simulink model "essai_echelon_volt"  (R2024a)
settings: Solver=VariableStepAuto  StartTime=0.0  StopTime=1000  RelTol=1e-3
InitFcn:
  | step_initial = get_param('simulink16marshihi/Échelon', 'Before');
  | set_param('simulink16marshihi/Température initiale', 'Value', step_initial);
  | set_param('simulink16marshihi/Chauffage/po_chauffage', 'Value', step_initial);
  | set_param('simulink16marshihi/Refroidissement/po_refroidissement', 'Value', step_initial);
  | consigne = get_param('simulink16marshihi/Échelon', 'After');
  | consigne = str2double(consigne);
  | step_initial = str2double(step_initial);
  | five_up = consigne + 0.05*abs(consigne-step_initial);
  | five_down = consigne - 0.05*abs(consigne-step_initial);
  | set_param('simulink16marshihi/+5%', 'Value', num2str(five_up));
  | set_param('simulink16marshihi/-5%', 'Value', num2str(five_down));
settings Model: Creator=sabri  LastModifiedBy=MADER143

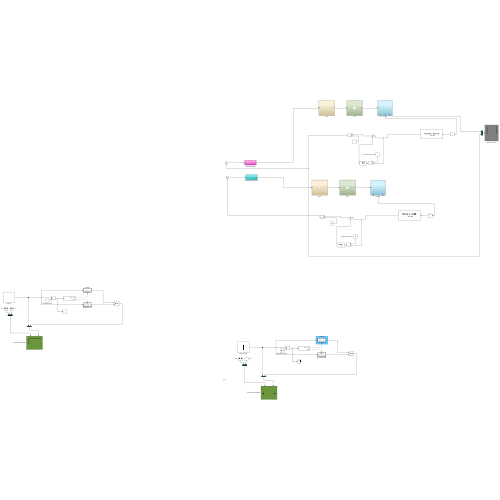
[thumbnail: Simulink's stored preview of the top-level diagram]
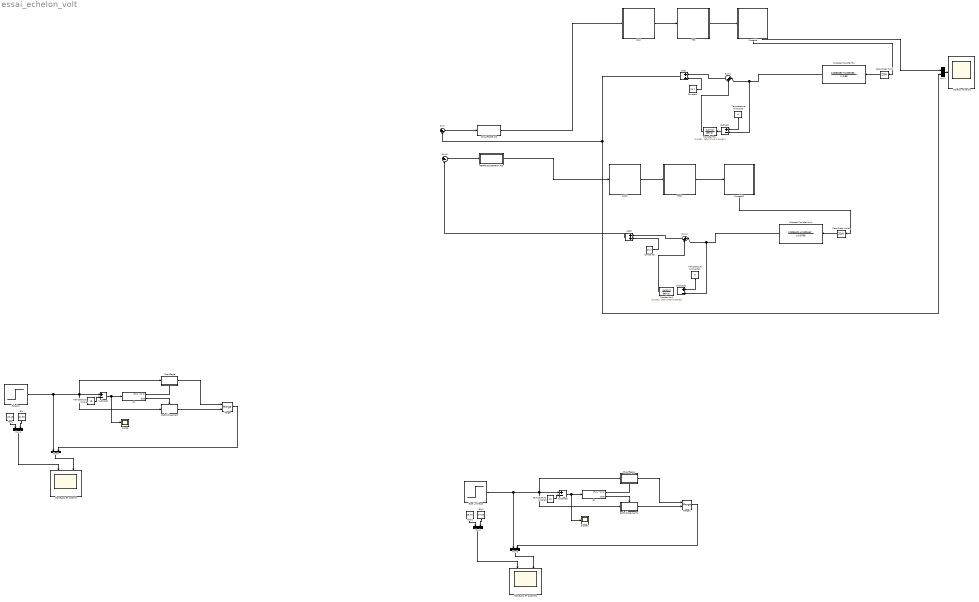
== system essai_echelon_volt ==
  " ÉCHELON ET SORTIE" : Scope  NumInputPorts=2
  " ÉCHELON ET SORTIE1" : Scope  NumInputPorts=2
  +5% : Constant  Value=25.45
  +5%1 : Constant  Value=25.45
  -5% : Constant  Value=24.55
  -5%1 : Constant  Value=24.55
  Add1 : Sum
  Add2 : Sum
  CHAUFFAGE PID : Subsystem
  Chauffage : Subsystem  TreatAsAtomicUnit=on
  Chauffage1 : Subsystem  TreatAsAtomicUnit=on
  Constant : Constant  Value=23.7
  Constant3 : Constant  Value=23.7
  DAC : Subsystem
  DAC1 : Subsystem
  Discrete Transfer Fcn : DiscreteTransferFcn  Numerator=[0.009158 0.009158]  Denominator=[1 -0.98]
  Discrete Transfer Fcn1 : DiscreteTransferFcn  Numerator=[0.009442 0.009442]  Denominator=[1 -0.9796]
  Essai_voltage : Step  Time=0  Before=16  After=25  SampleTime=0
  If1 : If  IfExpression=u1 >= 0
  If2 : If  IfExpression=u1 >= 0
  Merge : Merge
  Merge1 : Merge
  Mux{1..5} (5 alike) : Mux  Inputs=2
  Procédé : Subsystem
      settings: PortSchema="{\"entries\":[{\"content\":{\"sides\":[{\"content\":{\"connectorIds\":[\"In1\"]},\"type\":\"ConnectorPlacement.EquallySpacedRectSide\",\"uuid\":\"20a23230-a41b-4fdf-8ae4-039aa17abee7\"},{\"content\":{\"side\":\"RIGHT\"},\"type\":\"ConnectorPlacement.EquallySpacedRectSide\",\"uuid\":\"82e4e468-e0ad-4c9f-b6ff-cc9c1ee7ea9d\"},{\"content\":{\"side\":\"TOP\"},\"type\":\"ConnectorPlacement.EquallySpacedRectSide\",\"uuid\":\"049bc4af-9a9a-43aa-9803-dca862d69d2b\"},{\"content\":{\"connectorIds\":[\"Out1\",\"Out2\",\"Out3\"],\"side\":\"BOTTOM\"},\"type\":\"ConnectorPlacement.EquallySpacedRectSide\",\"uuid\":\"142d2b37-1c32-477b-9e70-4e4bc8b2913e\"}]},\"type\":\"ConnectorPlacement.EquallySpacedConnector\",\"uuid\":\"a0abf580-2deb-4a1c-9cb8-1272669a26fd\"}],\"packageUris\":[\"http://schema.mathworks.com/mf0/Connector/R2020b\"],\"version\":\"1.0\"}"
  Procédé1 : Subsystem
      settings: PortSchema="{\"entries\":[{\"content\":{\"sides\":[{\"content\":{\"connectorIds\":[\"In1\"]},\"type\":\"ConnectorPlacement.EquallySpacedRectSide\",\"uuid\":\"20a23230-a41b-4fdf-8ae4-039aa17abee7\"},{\"content\":{\"side\":\"RIGHT\"},\"type\":\"ConnectorPlacement.EquallySpacedRectSide\",\"uuid\":\"82e4e468-e0ad-4c9f-b6ff-cc9c1ee7ea9d\"},{\"content\":{\"side\":\"TOP\"},\"type\":\"ConnectorPlacement.EquallySpacedRectSide\",\"uuid\":\"049bc4af-9a9a-43aa-9803-dca862d69d2b\"},{\"content\":{\"connectorIds\":[\"Out1\",\"Out2\",\"Out3\"],\"side\":\"BOTTOM\"},\"type\":\"ConnectorPlacement.EquallySpacedRectSide\",\"uuid\":\"142d2b37-1c32-477b-9e70-4e4bc8b2913e\"}]},\"type\":\"ConnectorPlacement.EquallySpacedConnector\",\"uuid\":\"a0abf580-2deb-4a1c-9cb8-1272669a26fd\"}],\"packageUris\":[\"http://schema.mathworks.com/mf0/Connector/R2020b\"],\"version\":\"1.0\"}"
  REFROIDISSEMENT PID : Subsystem
  Refroidissement : Subsystem  TreatAsAtomicUnit=on
  Refroidissement1 : Subsystem  TreatAsAtomicUnit=on
  Scope : Scope
  Scope1 : Scope
  Subtract{,1..3} (4 alike) : Sum  Inputs=+-
  Sum : Sum  Inputs=|+-
  Sum1 : Sum  Inputs=|++
  Sum2 : Sum  Inputs=|++
  Sum3 : Sum  Inputs=|+-
  TEC : Subsystem
  TEC1 : Subsystem
  Température ambiante : Constant  Value=0
  Température ambiante1 : Constant  Value=0
  Température initiale : Constant  Value=16
  Température initiale1 : Constant  Value=16
  Transfer Fcn : TransferFcn  Numerator=[13.65]  Denominator=[900*2700*0.00161]
  Transfer Fcn1 : TransferFcn  Numerator=[13.65]  Denominator=[900*2700*0.00161]
  Zero-Order Hold : ZeroOrderHold  SampleTime=0.5
  Zero-Order Hold1 : ZeroOrderHold  SampleTime=0.5
  Échelon : Step  Time=0  Before=16  After=25  SampleTime=0
  Échelon et sortie : Scope
  wires:
  Échelon/1 -> Chauffage/1(In1), Subtract2/1, Refroidissement/1(In1), Mux5/1
  ? -> ?
  Température initiale/1 -> Subtract2/2
  +5%/1 -> Mux4/1
  -5%/1 -> Mux4/2
  If1/1 -> Chauffage/Action
  If1/2 -> Refroidissement/Action
  TEC1/1(W) -> Procédé1/1(W)
  DAC1/1(V) -> TEC1/1(V)
  Procédé1/2(y2) -> Zero-Order Hold1/1
  Température ambiante1/1 -> Subtract1/1
  Sum/1 -> CHAUFFAGE PID/1(In1)
  Sum2/1 -> Add2/1
  Add2/1 -> Sum3/2
  Sum3/1 -> REFROIDISSEMENT PID/1(In1)
  REFROIDISSEMENT PID/1(dc) -> DAC1/1(dc)
  Transfer Fcn1/1 -> Sum2/2
  Zero-Order Hold1/1 -> Discrete Transfer Fcn1/1
  Add1/1 -> Sum/2, Mux1/2
  Procédé/2(y2) -> Zero-Order Hold/1
  Zero-Order Hold/1 -> Discrete Transfer Fcn/1
  Subtract/1 -> Transfer Fcn/1
  Constant/1 -> Add1/2
  Discrete Transfer Fcn1/1 -> Sum2/1, Subtract1/2
  TEC/1(W) -> Procédé/1(W)
  CHAUFFAGE PID/1(dc) -> DAC/1(dc)
  Discrete Transfer Fcn/1 -> Sum1/1, Subtract/2
  Transfer Fcn/1 -> Sum1/2
  DAC/1(V) -> TEC/1(V)
  Sum1/1 -> Add1/1
  Constant3/1 -> Add2/2
  Procédé/3(y3) -> Mux1/1
  Température ambiante/1 -> Subtract/1
  Mux1/1 -> Échelon et sortie/1
  Chauffage/1(Out1) -> Merge/1
  Refroidissement/1(Out1) -> Merge/2
  Merge/1 -> Mux5/2
  Subtract2/1 -> Scope/1, If1/1
  Mux5/1 -> " ÉCHELON ET SORTIE"/2
  Mux4/1 -> " ÉCHELON ET SORTIE"/1
  Mux2/1 -> " ÉCHELON ET SORTIE1"/1
  Chauffage1/1(Out1) -> Merge1/1
  Mux3/1 -> " ÉCHELON ET SORTIE1"/2
  Refroidissement1/1(Out1) -> Merge1/2
  Merge1/1 -> Mux3/2
  Subtract3/1 -> Scope1/1, If2/1
  If2/2 -> Refroidissement1/Action
  If2/1 -> Chauffage1/Action
  +5%1/1 -> Mux2/1
  Température initiale1/1 -> Subtract3/2
  -5%1/1 -> Mux2/2
  Essai_voltage/1 -> Chauffage1/1(In1), Subtract3/1, Refroidissement1/1(In1), Mux3/1

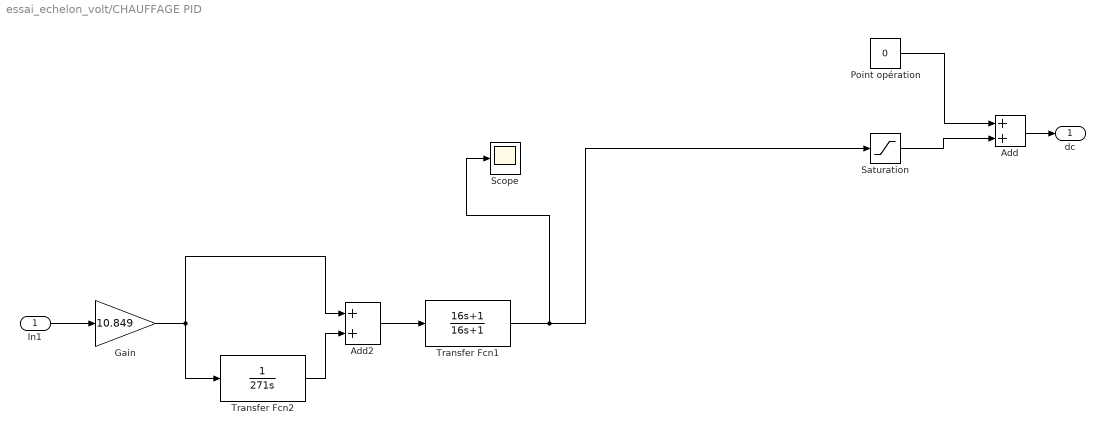
== system essai_echelon_volt/CHAUFFAGE PID ==
  In1 : Inport
  Add : Sum
  Add2 : Sum
  Gain : Gain  Gain=10.849
  Point opération : Constant  Value=0
  Saturation : Saturate  UpperLimit=255  LowerLimit=-255
  Scope : Scope
  Transfer Fcn1 : TransferFcn  Numerator=[16 1]  Denominator=[16 1]
  Transfer Fcn2 : TransferFcn  Denominator=[271 0]
  dc : Outport
  wires:
  Add2/1 -> Transfer Fcn1/1
  Saturation/1 -> Add/2
  Point opération/1 -> Add/1
  Transfer Fcn1/1 -> Scope/1, Saturation/1
  Gain/1 -> Transfer Fcn2/1, Add2/1
  Transfer Fcn2/1 -> Add2/2
  In1/1 -> Gain/1
  Add/1 -> dc/1

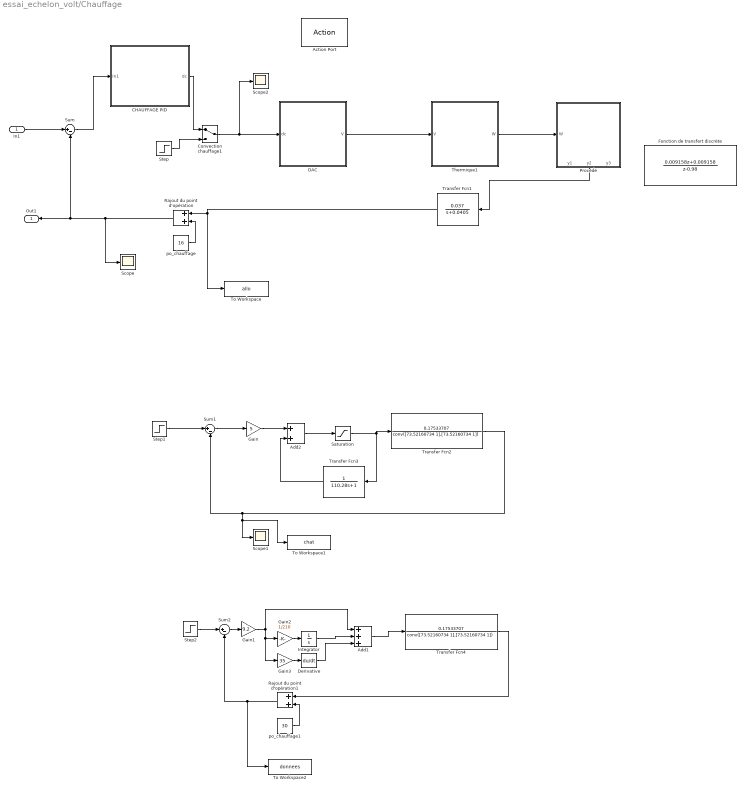
== system essai_echelon_volt/Chauffage ==
  In1 : Inport
  Action Port : ActionPort  ActionPortLabel=if(u1 >= 0)
  Add1 : Sum  Inputs=+++
  Add2 : Sum
  CHAUFFAGE PID : Subsystem
  Convection chauffage1 : ManualSwitch
  DAC : Subsystem
  Derivative : Derivative
  Fonction de transfert discrète : DiscreteTransferFcn  Numerator=[0.009158 0.009158]  Denominator=[1 -0.98]
  Gain : Gain  Gain=5
  Gain1 : Gain  Gain=9.2
  Gain2 : Gain  Gain=1/210
  Gain3 : Gain  Gain=35
  Integrator : Integrator
  Procédé : Subsystem
      settings: PortSchema="{\"entries\":[{\"content\":{\"sides\":[{\"content\":{\"connectorIds\":[\"In1\"]},\"type\":\"ConnectorPlacement.EquallySpacedRectSide\",\"uuid\":\"20a23230-a41b-4fdf-8ae4-039aa17abee7\"},{\"content\":{\"side\":\"RIGHT\"},\"type\":\"ConnectorPlacement.EquallySpacedRectSide\",\"uuid\":\"82e4e468-e0ad-4c9f-b6ff-cc9c1ee7ea9d\"},{\"content\":{\"side\":\"TOP\"},\"type\":\"ConnectorPlacement.EquallySpacedRectSide\",\"uuid\":\"049bc4af-9a9a-43aa-9803-dca862d69d2b\"},{\"content\":{\"connectorIds\":[\"Out1\",\"Out2\",\"Out3\"],\"side\":\"BOTTOM\"},\"type\":\"ConnectorPlacement.EquallySpacedRectSide\",\"uuid\":\"142d2b37-1c32-477b-9e70-4e4bc8b2913e\"}]},\"type\":\"ConnectorPlacement.EquallySpacedConnector\",\"uuid\":\"a0abf580-2deb-4a1c-9cb8-1272669a26fd\"}],\"packageUris\":[\"http://schema.mathworks.com/mf0/Connector/R2020b\"],\"version\":\"1.0\"}"
  Rajout du point d'opération : Sum
  Rajout du point d'opération1 : Sum
  Saturation : Saturate  UpperLimit=100  LowerLimit=-100
  Scope : Scope
  Scope1 : Scope
  Scope2 : Scope
  Step : Step  Time=0  After=20  SampleTime=0
  Step1 : Step  Time=0  After=7  SampleTime=0
  Step2 : Step  Time=0  Before=23  After=30  SampleTime=0
  Sum : Sum  Inputs=|+-
  Sum1 : Sum  Inputs=|+-
  Sum2 : Sum  Inputs=|+-
  Thermique1 : Subsystem
  To Workspace : ToWorkspace  VariableName=allo  SampleTime=-1
  To Workspace1 : ToWorkspace  VariableName=chat  SampleTime=-1
  To Workspace2 : ToWorkspace  VariableName=donnees  SampleTime=-1
  Transfer Fcn1 : TransferFcn  Numerator=[0.037]  Denominator=[1 0.0405]
  Transfer Fcn2 : TransferFcn  Numerator=[0.17533707]  Denominator=conv([73.52160734 1],[73.52160734 1])
  Transfer Fcn3 : TransferFcn  Denominator=[110.28 1]
  Transfer Fcn4 : TransferFcn  Numerator=[0.17533707]  Denominator=conv([73.52160734 1],[73.52160734 1])
  po_chauffage : Constant  Value=16
  po_chauffage1 : Constant  Value=30
  Out1 : Outport
  wires:
  Sum/1 -> CHAUFFAGE PID/1(In1)
  In1/1 -> Sum/1
  Rajout du point d'opération/1 -> Scope/1, Out1/1, Sum/2
  po_chauffage/1 -> Rajout du point d'opération/2
  Procédé/2(y2) -> Transfer Fcn1/1
  Transfer Fcn1/1 -> To Workspace/1, Rajout du point d'opération/1
  DAC/1(V) -> Thermique1/1(V)
  CHAUFFAGE PID/1(dc) -> Convection chauffage1/1
  Convection chauffage1/1 -> Scope2/1, DAC/1(dc)
  Step/1 -> Convection chauffage1/2
  Step1/1 -> Sum1/1
  Transfer Fcn2/1 -> To Workspace1/1, Scope1/1, Sum1/2
  Gain/1 -> Add2/1
  Transfer Fcn3/1 -> Add2/2
  Add2/1 -> Saturation/1
  Saturation/1 -> Transfer Fcn2/1, Transfer Fcn3/1
  Sum1/1 -> Gain/1
  Thermique1/1(W) -> Procédé/1(W)
  Gain2/1 -> Integrator/1
  Add1/1 -> Transfer Fcn4/1
  Gain3/1 -> Derivative/1
  Sum2/1 -> Gain1/1
  Integrator/1 -> Add1/2
  Derivative/1 -> Add1/3
  Gain1/1 -> Add1/1, Gain3/1, Gain2/1
  Rajout du point d'opération1/1 -> To Workspace2/1, Sum2/2
  Transfer Fcn4/1 -> Rajout du point d'opération1/1
  po_chauffage1/1 -> Rajout du point d'opération1/2
  Step2/1 -> Sum2/1

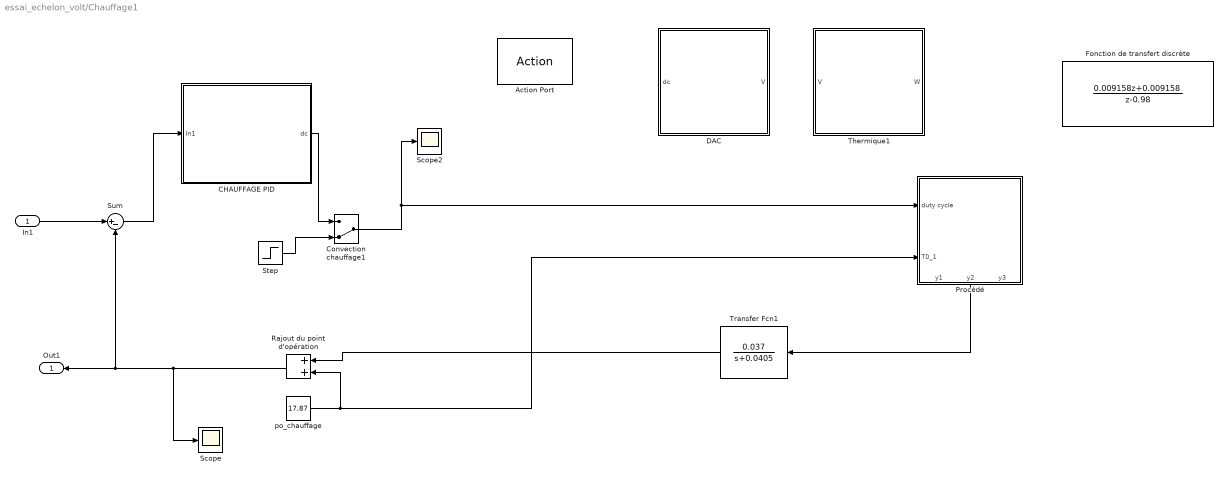
== system essai_echelon_volt/Chauffage1 ==
  In1 : Inport
  Action Port : ActionPort  ActionPortLabel=if(u1 >= 0)
  CHAUFFAGE PID : Subsystem
  Convection chauffage1 : ManualSwitch  CurrentSetting=0
  DAC : Subsystem
  Fonction de transfert discrète : DiscreteTransferFcn  Numerator=[0.009158 0.009158]  Denominator=[1 -0.98]
  Procédé : Subsystem
      settings: PortSchema="{\"entries\":[{\"content\":{\"sides\":[{\"content\":{\"connectorIds\":[\"In1\",\"In2\"]},\"type\":\"ConnectorPlacement.EquallySpacedRectSide\",\"uuid\":\"20a23230-a41b-4fdf-8ae4-039aa17abee7\"},{\"content\":{\"side\":\"RIGHT\"},\"type\":\"ConnectorPlacement.EquallySpacedRectSide\",\"uuid\":\"82e4e468-e0ad-4c9f-b6ff-cc9c1ee7ea9d\"},{\"content\":{\"side\":\"TOP\"},\"type\":\"ConnectorPlacement.EquallySpacedRectSide\",\"uuid\":\"049bc4af-9a9a-43aa-9803-dca862d69d2b\"},{\"content\":{\"connectorIds\":[\"Out1\",\"Out2\",\"Out3\"],\"side\":\"BOTTOM\"},\"type\":\"ConnectorPlacement.EquallySpacedRectSide\",\"uuid\":\"142d2b37-1c32-477b-9e70-4e4bc8b2913e\"}]},\"type\":\"ConnectorPlacement.EquallySpacedConnector\",\"uuid\":\"a0abf580-2deb-4a1c-9cb8-1272669a26fd\"}],\"packageUris\":[\"http://schema.mathworks.com/mf0/Connector/R2020b\"],\"version\":\"1.0\"}"
  Rajout du point d'opération : Sum
  Scope : Scope
  Scope2 : Scope
  Step : Step  Time=0  After=3.92  SampleTime=0
  Sum : Sum  Inputs=|+-
  Thermique1 : Subsystem
  Transfer Fcn1 : TransferFcn  Numerator=[0.037]  Denominator=[1 0.0405]
  po_chauffage : Constant  Value=17.87
  Out1 : Outport
  wires:
  Sum/1 -> CHAUFFAGE PID/1(In1)
  In1/1 -> Sum/1
  Rajout du point d'opération/1 -> Scope/1, Out1/1, Sum/2
  po_chauffage/1 -> Procédé/2(T0_1), Rajout du point d'opération/2
  Procédé/2(y2) -> Transfer Fcn1/1
  Transfer Fcn1/1 -> Rajout du point d'opération/1
  CHAUFFAGE PID/1(dc) -> Convection chauffage1/1
  Convection chauffage1/1 -> Procédé/1(duty cycle), Scope2/1
  Step/1 -> Convection chauffage1/2

== system essai_echelon_volt/DAC ==
  dc : Inport
  Slope : Gain  Gain=0.079
  V : Outport
  wires:
  dc/1 -> Slope/1
  Slope/1 -> V/1

== system essai_echelon_volt/DAC1 ==
  dc : Inport
  Slope : Gain  Gain=0.079
  V : Outport
  wires:
  dc/1 -> Slope/1
  Slope/1 -> V/1

== system essai_echelon_volt/Procédé ==
  W : Inport
  Add : Sum
  G1 : TransferFcn  Numerator=[0.006923]  Denominator=[1 0.01236]
  G2 : TransferFcn  Numerator=[0.01782]  Denominator=[1 0.02491]
  G3 : TransferFcn  Numerator=[0.037]  Denominator=[1 0.0405]
  Step : Step  Time=60  After=0  SampleTime=0
  y1 : Outport
  y2 : Outport  Port=2
  y3 : Outport  Port=3
  wires:
  G1/1 -> y1/1, G2/1
  Add/1 -> G1/1
  W/1 -> Add/1
  Step/1 -> Add/2
  G2/1 -> G3/1, y2/1
  G3/1 -> y3/1

== system essai_echelon_volt/Procédé1 ==
  W : Inport
  Add : Sum
  G1 : TransferFcn  Numerator=[0.009117]  Denominator=[1 0.01046]
  G2 : TransferFcn  Numerator=[0.03203]  Denominator=[1 0.03834]
  G3 : TransferFcn  Numerator=[0.03816]  Denominator=[1 0.04131]
  Step : Step  Time=60  After=0  SampleTime=0
  y1 : Outport
  y2 : Outport  Port=2
  y3 : Outport  Port=3
  wires:
  G1/1 -> y1/1, G2/1
  Add/1 -> G1/1
  W/1 -> Add/1
  Step/1 -> Add/2
  G2/1 -> G3/1, y2/1
  G3/1 -> y3/1

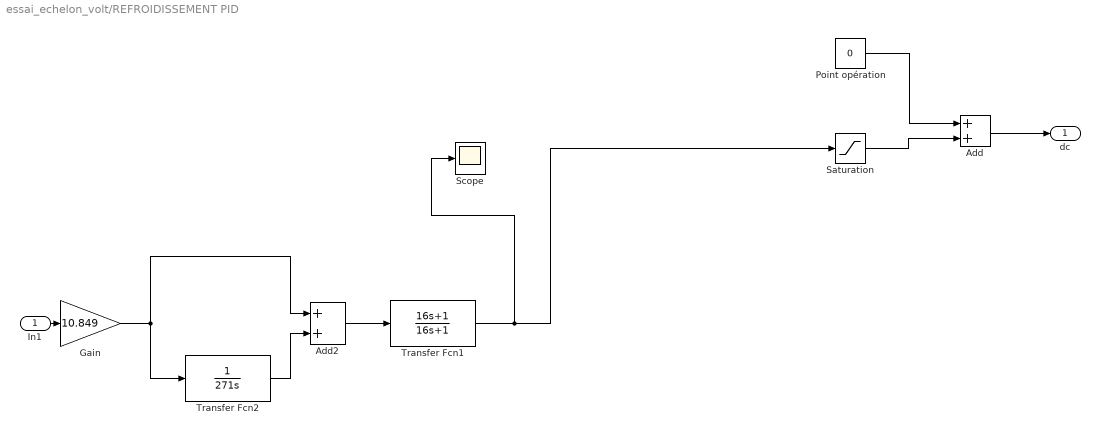
== system essai_echelon_volt/REFROIDISSEMENT PID ==
  In1 : Inport
  Add : Sum
  Add2 : Sum
  Gain : Gain  Gain=10.849
  Point opération : Constant  Value=0
  Saturation : Saturate  UpperLimit=255  LowerLimit=-255
  Scope : Scope
  Transfer Fcn1 : TransferFcn  Numerator=[16 1]  Denominator=[16 1]
  Transfer Fcn2 : TransferFcn  Denominator=[271 0]
  dc : Outport
  wires:
  Add2/1 -> Transfer Fcn1/1
  Saturation/1 -> Add/2
  Point opération/1 -> Add/1
  Transfer Fcn1/1 -> Scope/1, Saturation/1
  Gain/1 -> Transfer Fcn2/1, Add2/1
  Transfer Fcn2/1 -> Add2/2
  In1/1 -> Gain/1
  Add/1 -> dc/1

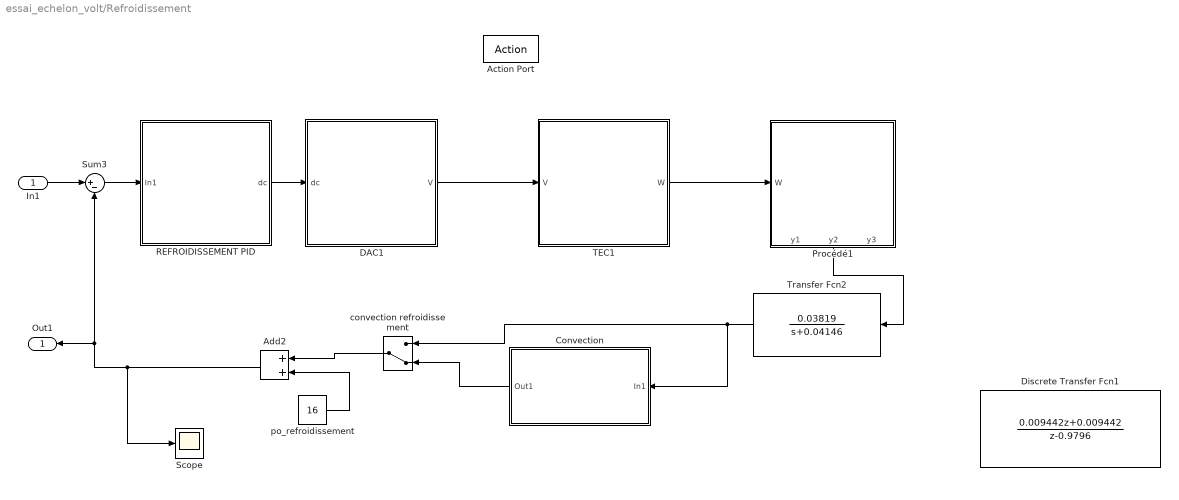
== system essai_echelon_volt/Refroidissement ==
  In1 : Inport
  Action Port : ActionPort  ActionPortLabel=else
  Add2 : Sum
  Convection : Subsystem
  DAC1 : Subsystem
  Discrete Transfer Fcn1 : DiscreteTransferFcn  Numerator=[0.009442 0.009442]  Denominator=[1 -0.9796]
  Procédé1 : Subsystem
      settings: PortSchema="{\"entries\":[{\"content\":{\"sides\":[{\"content\":{\"connectorIds\":[\"In1\"]},\"type\":\"ConnectorPlacement.EquallySpacedRectSide\",\"uuid\":\"20a23230-a41b-4fdf-8ae4-039aa17abee7\"},{\"content\":{\"side\":\"RIGHT\"},\"type\":\"ConnectorPlacement.EquallySpacedRectSide\",\"uuid\":\"82e4e468-e0ad-4c9f-b6ff-cc9c1ee7ea9d\"},{\"content\":{\"side\":\"TOP\"},\"type\":\"ConnectorPlacement.EquallySpacedRectSide\",\"uuid\":\"049bc4af-9a9a-43aa-9803-dca862d69d2b\"},{\"content\":{\"connectorIds\":[\"Out1\",\"Out2\",\"Out3\"],\"side\":\"BOTTOM\"},\"type\":\"ConnectorPlacement.EquallySpacedRectSide\",\"uuid\":\"142d2b37-1c32-477b-9e70-4e4bc8b2913e\"}]},\"type\":\"ConnectorPlacement.EquallySpacedConnector\",\"uuid\":\"a0abf580-2deb-4a1c-9cb8-1272669a26fd\"}],\"packageUris\":[\"http://schema.mathworks.com/mf0/Connector/R2020b\"],\"version\":\"1.0\"}"
  REFROIDISSEMENT PID : Subsystem
  Scope : Scope
  Sum3 : Sum  Inputs=|+-
  TEC1 : Subsystem
  Transfer Fcn2 : TransferFcn  Numerator=[0.03819]  Denominator=[1 0.04146]
  convection refroidissement : ManualSwitch  CurrentSetting=0
  po_refroidissement : Constant  Value=16
  Out1 : Outport
  wires:
  TEC1/1(W) -> Procédé1/1(W)
  DAC1/1(V) -> TEC1/1(V)
  Procédé1/2(y2) -> Transfer Fcn2/1
  po_refroidissement/1 -> Add2/2
  Add2/1 -> Scope/1, Out1/1, Sum3/2
  Sum3/1 -> REFROIDISSEMENT PID/1(In1)
  REFROIDISSEMENT PID/1(dc) -> DAC1/1(dc)
  In1/1 -> Sum3/1
  Transfer Fcn2/1 -> Convection/1(In1), convection refroidissement/1
  convection refroidissement/1 -> Add2/1
  Convection/1(Out1) -> convection refroidissement/2

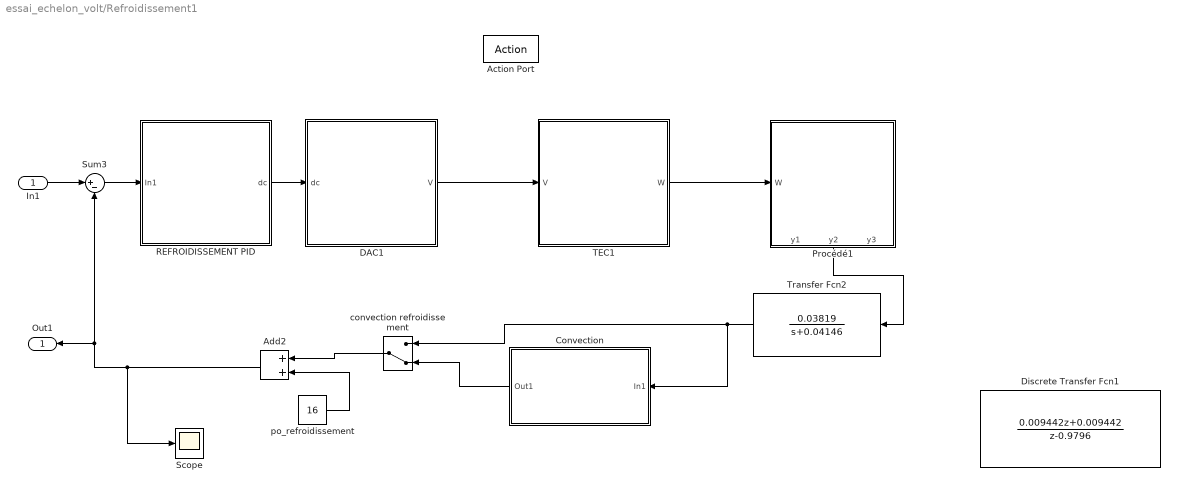
== system essai_echelon_volt/Refroidissement1 ==
  In1 : Inport
  Action Port : ActionPort  ActionPortLabel=else
  Add2 : Sum
  Convection : Subsystem
  DAC1 : Subsystem
  Discrete Transfer Fcn1 : DiscreteTransferFcn  Numerator=[0.009442 0.009442]  Denominator=[1 -0.9796]
  Procédé1 : Subsystem
      settings: PortSchema="{\"entries\":[{\"content\":{\"sides\":[{\"content\":{\"connectorIds\":[\"In1\"]},\"type\":\"ConnectorPlacement.EquallySpacedRectSide\",\"uuid\":\"20a23230-a41b-4fdf-8ae4-039aa17abee7\"},{\"content\":{\"side\":\"RIGHT\"},\"type\":\"ConnectorPlacement.EquallySpacedRectSide\",\"uuid\":\"82e4e468-e0ad-4c9f-b6ff-cc9c1ee7ea9d\"},{\"content\":{\"side\":\"TOP\"},\"type\":\"ConnectorPlacement.EquallySpacedRectSide\",\"uuid\":\"049bc4af-9a9a-43aa-9803-dca862d69d2b\"},{\"content\":{\"connectorIds\":[\"Out1\",\"Out2\",\"Out3\"],\"side\":\"BOTTOM\"},\"type\":\"ConnectorPlacement.EquallySpacedRectSide\",\"uuid\":\"142d2b37-1c32-477b-9e70-4e4bc8b2913e\"}]},\"type\":\"ConnectorPlacement.EquallySpacedConnector\",\"uuid\":\"a0abf580-2deb-4a1c-9cb8-1272669a26fd\"}],\"packageUris\":[\"http://schema.mathworks.com/mf0/Connector/R2020b\"],\"version\":\"1.0\"}"
  REFROIDISSEMENT PID : Subsystem
  Scope : Scope
  Sum3 : Sum  Inputs=|+-
  TEC1 : Subsystem
  Transfer Fcn2 : TransferFcn  Numerator=[0.03819]  Denominator=[1 0.04146]
  convection refroidissement : ManualSwitch  CurrentSetting=0
  po_refroidissement : Constant  Value=16
  Out1 : Outport
  wires:
  TEC1/1(W) -> Procédé1/1(W)
  DAC1/1(V) -> TEC1/1(V)
  Procédé1/2(y2) -> Transfer Fcn2/1
  po_refroidissement/1 -> Add2/2
  Add2/1 -> Scope/1, Out1/1, Sum3/2
  Sum3/1 -> REFROIDISSEMENT PID/1(In1)
  REFROIDISSEMENT PID/1(dc) -> DAC1/1(dc)
  In1/1 -> Sum3/1
  Transfer Fcn2/1 -> Convection/1(In1), convection refroidissement/1
  convection refroidissement/1 -> Add2/1
  Convection/1(Out1) -> convection refroidissement/2

== system essai_echelon_volt/TEC ==
  V : Inport
  MATLAB Function : MATLAB Function  TreatAsAtomicUnit=on
  W : Outport
  wires:
  V/1 -> MATLAB Function/1(u)
  MATLAB Function/1(y) -> W/1

== system essai_echelon_volt/TEC1 ==
  V : Inport
  MATLAB Function : MATLAB Function  TreatAsAtomicUnit=on
  W : Outport
  wires:
  V/1 -> MATLAB Function/1(u)
  MATLAB Function/1(y) -> W/1

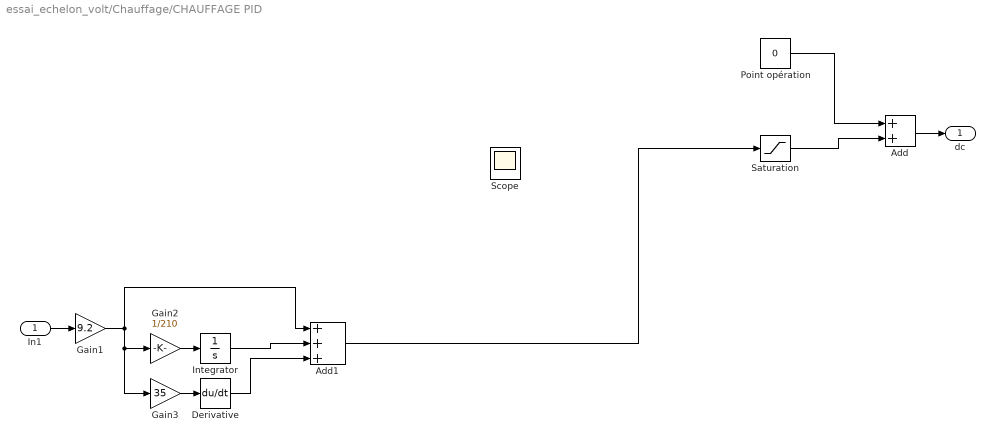
== system essai_echelon_volt/Chauffage/CHAUFFAGE PID ==
  In1 : Inport
  Add : Sum
  Add1 : Sum  Inputs=+++
  Derivative : Derivative
  Gain1 : Gain  Gain=9.2
  Gain2 : Gain  Gain=1/210
  Gain3 : Gain  Gain=35
  Integrator : Integrator
  Point opération : Constant  Value=0
  Saturation : Saturate  UpperLimit=100  LowerLimit=-100  LinearizeAsGain=off
  Scope : Scope
  dc : Outport
  wires:
  Saturation/1 -> Add/2
  Point opération/1 -> Add/1
  Add/1 -> dc/1
  Derivative/1 -> Add1/3
  In1/1 -> Gain1/1
  Gain3/1 -> Derivative/1
  Integrator/1 -> Add1/2
  Gain1/1 -> Add1/1, Gain3/1, Gain2/1
  Gain2/1 -> Integrator/1
  Add1/1 -> Saturation/1

== system essai_echelon_volt/Chauffage/DAC ==
  dc : Inport
  Slope : Gain  Gain=0.079
  V : Outport
  wires:
  dc/1 -> Slope/1
  Slope/1 -> V/1

== system essai_echelon_volt/Chauffage/Procédé ==
  W : Inport
  Add : Sum
  G1 : TransferFcn  Numerator=[0.01775]  Denominator=[1 0.01236]
  G2 : TransferFcn  Numerator=[0.01782]  Denominator=[1 0.02491]
  G3 : TransferFcn  Numerator=[0.037]  Denominator=[1 0.0405]
  Step : Step  Time=60  After=0  SampleTime=0
  y1 : Outport
  y2 : Outport  Port=2
  y3 : Outport  Port=3
  wires:
  G1/1 -> y1/1, G2/1
  Add/1 -> G1/1
  W/1 -> Add/1
  Step/1 -> Add/2
  G2/1 -> G3/1, y2/1
  G3/1 -> y3/1

== system essai_echelon_volt/Chauffage/Thermique1 ==
  V : Inport
  MATLAB Function : MATLAB Function  TreatAsAtomicUnit=on
  W : Outport
  wires:
  V/1 -> MATLAB Function/1(u)
  MATLAB Function/1(y) -> W/1

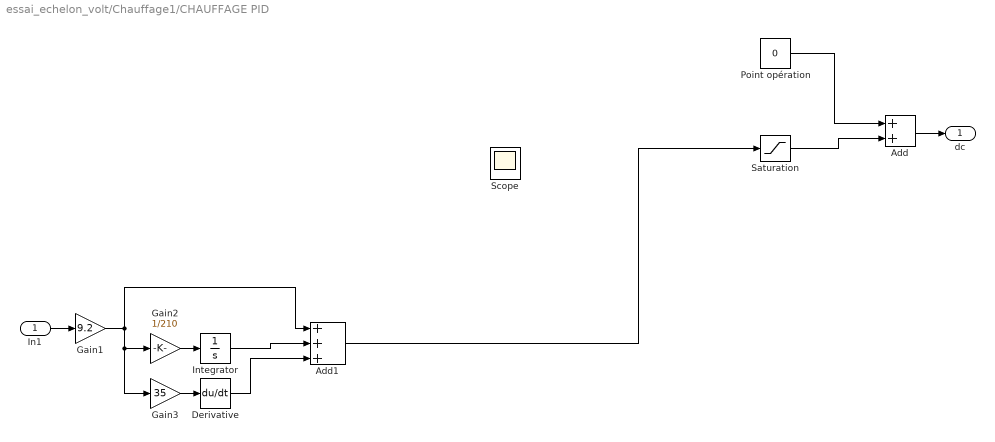
== system essai_echelon_volt/Chauffage1/CHAUFFAGE PID ==
  In1 : Inport
  Add : Sum
  Add1 : Sum  Inputs=+++
  Derivative : Derivative
  Gain1 : Gain  Gain=9.2
  Gain2 : Gain  Gain=1/210
  Gain3 : Gain  Gain=35
  Integrator : Integrator
  Point opération : Constant  Value=0
  Saturation : Saturate  UpperLimit=100  LowerLimit=-100  LinearizeAsGain=off
  Scope : Scope
  dc : Outport
  wires:
  Saturation/1 -> Add/2
  Point opération/1 -> Add/1
  Add/1 -> dc/1
  Derivative/1 -> Add1/3
  In1/1 -> Gain1/1
  Gain3/1 -> Derivative/1
  Integrator/1 -> Add1/2
  Gain1/1 -> Add1/1, Gain3/1, Gain2/1
  Gain2/1 -> Integrator/1
  Add1/1 -> Saturation/1

== system essai_echelon_volt/Chauffage1/DAC ==
  dc : Inport
  Slope : Gain  Gain=0.079
  V : Outport
  wires:
  dc/1 -> Slope/1
  Slope/1 -> V/1

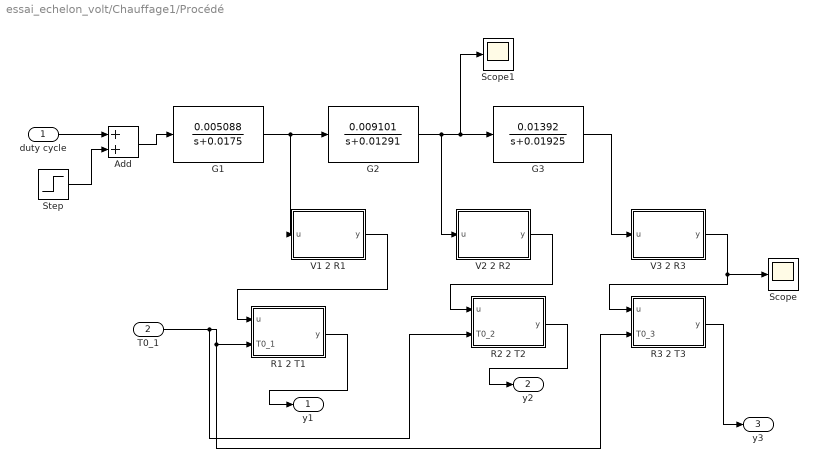
== system essai_echelon_volt/Chauffage1/Procédé ==
  duty cycle : Inport
  T0_1 : Inport  Port=2
  Add : Sum
  G1 : TransferFcn  Numerator=[0.005088]  Denominator=[1 0.0175]
  G2 : TransferFcn  Numerator=[0.009101]  Denominator=[1 0.01291]
  G3 : TransferFcn  Numerator=[0.01392]  Denominator=[1 0.01925]
  R1 2 T1 : MATLAB Function  TreatAsAtomicUnit=on
  R2 2 T2 : MATLAB Function  TreatAsAtomicUnit=on
  R3 2 T3 : MATLAB Function  TreatAsAtomicUnit=on
  Scope : Scope
  Scope1 : Scope
  Step : Step  Time=60  After=0  SampleTime=0
  V1 2 R1 : MATLAB Function  TreatAsAtomicUnit=on
  V2 2 R2 : MATLAB Function  TreatAsAtomicUnit=on
  V3 2 R3 : MATLAB Function  TreatAsAtomicUnit=on
  y1 : Outport
  y2 : Outport  Port=2
  y3 : Outport  Port=3
  wires:
  G1/1 -> V1 2 R1/1(u), G2/1
  Add/1 -> G1/1
  duty cycle/1 -> Add/1
  Step/1 -> Add/2
  G3/1 -> V3 2 R3/1(u)
  V1 2 R1/1(y) -> R1 2 T1/1(u)
  R1 2 T1/1(y) -> y1/1
  V2 2 R2/1(y) -> R2 2 T2/1(u)
  R2 2 T2/1(y) -> y2/1
  V3 2 R3/1(y) -> Scope/1, R3 2 T3/1(u)
  R3 2 T3/1(y) -> y3/1
  T0_1/1 -> R2 2 T2/2(T0_2), R3 2 T3/2(T0_3), R1 2 T1/2(T0_1)
  G2/1 -> V2 2 R2/1(u), Scope1/1, G3/1

== system essai_echelon_volt/Chauffage1/Thermique1 ==
  V : Inport
  MATLAB Function : MATLAB Function  TreatAsAtomicUnit=on
  W : Outport
  wires:
  V/1 -> MATLAB Function/1(u)
  MATLAB Function/1(y) -> W/1

== system essai_echelon_volt/Refroidissement/Convection ==
  In1 : Inport
  Subtract1 : Sum  Inputs=+-
  Sum2 : Sum  Inputs=|++
  Transfer Fcn1 : TransferFcn  Numerator=[13.65]  Denominator=[900*2700*0.00161]
  point d'opération : Constant  Value=0
  Out1 : Outport
  wires:
  Sum2/1 -> Out1/1
  In1/1 -> Subtract1/2, Sum2/1
  point d'opération/1 -> Subtract1/1
  Subtract1/1 -> Transfer Fcn1/1
  Transfer Fcn1/1 -> Sum2/2

== system essai_echelon_volt/Refroidissement/DAC1 ==
  dc : Inport
  Slope : Gain  Gain=0.079
  V : Outport
  wires:
  dc/1 -> Slope/1
  Slope/1 -> V/1

== system essai_echelon_volt/Refroidissement/Procédé1 ==
  W : Inport
  Add : Sum
  G1 : TransferFcn  Numerator=[0.009117]  Denominator=[1 0.01046]
  G2 : TransferFcn  Numerator=[0.03203]  Denominator=[1 0.03834]
  G3 : TransferFcn  Numerator=[0.03816]  Denominator=[1 0.04131]
  Step : Step  Time=60  After=0  SampleTime=0
  y1 : Outport
  y2 : Outport  Port=2
  y3 : Outport  Port=3
  wires:
  G1/1 -> y1/1, G2/1
  Add/1 -> G1/1
  W/1 -> Add/1
  Step/1 -> Add/2
  G2/1 -> G3/1, y2/1
  G3/1 -> y3/1

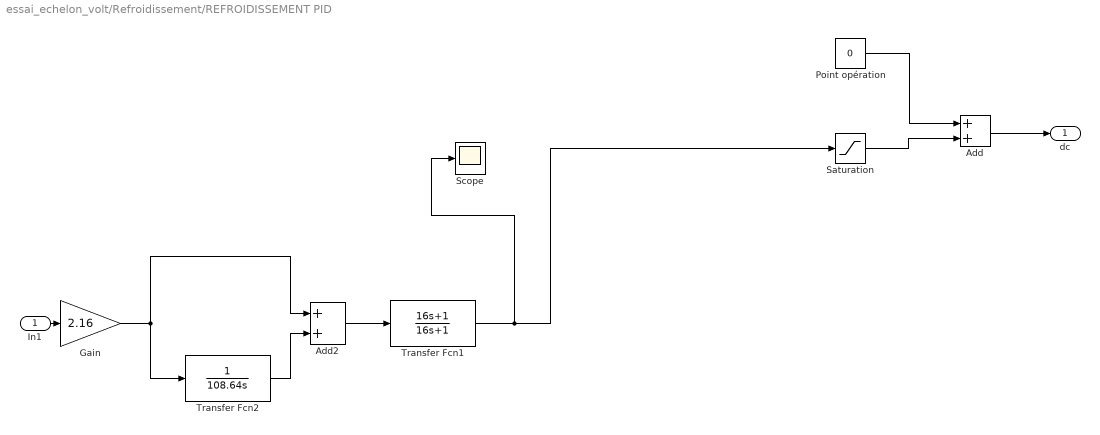
== system essai_echelon_volt/Refroidissement/REFROIDISSEMENT PID ==
  In1 : Inport
  Add : Sum
  Add2 : Sum
  Gain : Gain  Gain=2.16
  Point opération : Constant  Value=0
  Saturation : Saturate  UpperLimit=255  LowerLimit=-255
  Scope : Scope
  Transfer Fcn1 : TransferFcn  Numerator=[16 1]  Denominator=[16 1]
  Transfer Fcn2 : TransferFcn  Denominator=[108.64 0]
  dc : Outport
  wires:
  Add2/1 -> Transfer Fcn1/1
  Saturation/1 -> Add/2
  Point opération/1 -> Add/1
  Transfer Fcn1/1 -> Scope/1, Saturation/1
  Gain/1 -> Transfer Fcn2/1, Add2/1
  Transfer Fcn2/1 -> Add2/2
  In1/1 -> Gain/1
  Add/1 -> dc/1

== system essai_echelon_volt/Refroidissement/TEC1 ==
  V : Inport
  MATLAB Function : MATLAB Function  TreatAsAtomicUnit=on
  W : Outport
  wires:
  V/1 -> MATLAB Function/1(u)
  MATLAB Function/1(y) -> W/1

== system essai_echelon_volt/Refroidissement1/Convection ==
  In1 : Inport
  Subtract1 : Sum  Inputs=+-
  Sum2 : Sum  Inputs=|++
  Transfer Fcn1 : TransferFcn  Numerator=[13.65]  Denominator=[900*2700*0.00161]
  point d'opération : Constant  Value=0
  Out1 : Outport
  wires:
  Sum2/1 -> Out1/1
  In1/1 -> Subtract1/2, Sum2/1
  point d'opération/1 -> Subtract1/1
  Subtract1/1 -> Transfer Fcn1/1
  Transfer Fcn1/1 -> Sum2/2

== system essai_echelon_volt/Refroidissement1/DAC1 ==
  dc : Inport
  Slope : Gain  Gain=0.079
  V : Outport
  wires:
  dc/1 -> Slope/1
  Slope/1 -> V/1

== system essai_echelon_volt/Refroidissement1/Procédé1 ==
  W : Inport
  Add : Sum
  G1 : TransferFcn  Numerator=[0.009117]  Denominator=[1 0.01046]
  G2 : TransferFcn  Numerator=[0.03203]  Denominator=[1 0.03834]
  G3 : TransferFcn  Numerator=[0.03816]  Denominator=[1 0.04131]
  Step : Step  Time=60  After=0  SampleTime=0
  y1 : Outport
  y2 : Outport  Port=2
  y3 : Outport  Port=3
  wires:
  G1/1 -> y1/1, G2/1
  Add/1 -> G1/1
  W/1 -> Add/1
  Step/1 -> Add/2
  G2/1 -> G3/1, y2/1
  G3/1 -> y3/1

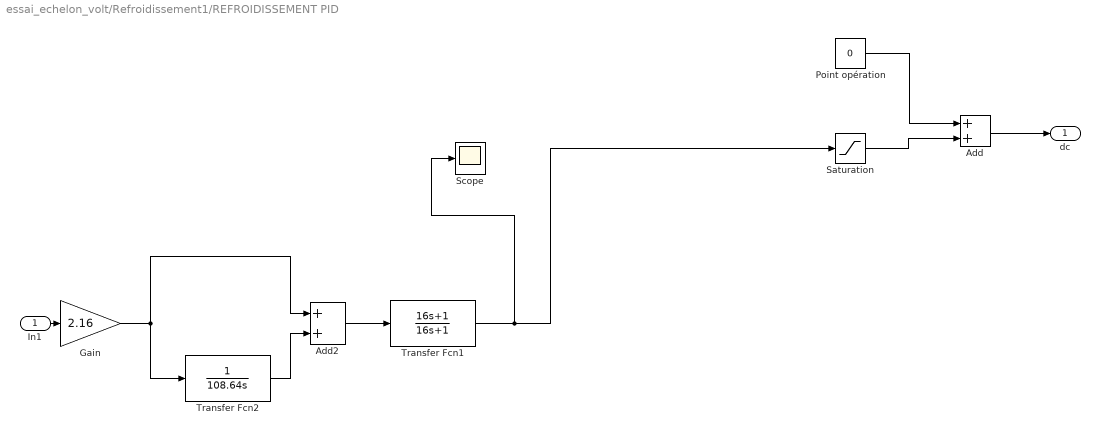
== system essai_echelon_volt/Refroidissement1/REFROIDISSEMENT PID ==
  In1 : Inport
  Add : Sum
  Add2 : Sum
  Gain : Gain  Gain=2.16
  Point opération : Constant  Value=0
  Saturation : Saturate  UpperLimit=255  LowerLimit=-255
  Scope : Scope
  Transfer Fcn1 : TransferFcn  Numerator=[16 1]  Denominator=[16 1]
  Transfer Fcn2 : TransferFcn  Denominator=[108.64 0]
  dc : Outport
  wires:
  Add2/1 -> Transfer Fcn1/1
  Saturation/1 -> Add/2
  Point opération/1 -> Add/1
  Transfer Fcn1/1 -> Scope/1, Saturation/1
  Gain/1 -> Transfer Fcn2/1, Add2/1
  Transfer Fcn2/1 -> Add2/2
  In1/1 -> Gain/1
  Add/1 -> dc/1

== system essai_echelon_volt/Refroidissement1/TEC1 ==
  V : Inport
  MATLAB Function : MATLAB Function  TreatAsAtomicUnit=on
  W : Outport
  wires:
  V/1 -> MATLAB Function/1(u)
  MATLAB Function/1(y) -> W/1

== matlab function essai_echelon_volt/TEC1/MATLAB Function ==
  data: u input; y output
function y = fcn(u)
y=6.15*u;

== matlab function essai_echelon_volt/TEC/MATLAB Function ==
  data: u input; y output
function y = fcn(u)
y=6.15*u;

== matlab function essai_echelon_volt/Chauffage1/Thermique1/MATLAB Function ==
  data: u input; y output
function y = fcn(u)
y=0.9089*u*u+0.19711*u;

== matlab function essai_echelon_volt/Refroidissement/TEC1/MATLAB Function ==
  data: u input; y output
function y = fcn(u)
y=6.15*u;

== matlab function essai_echelon_volt/Chauffage/Thermique1/MATLAB Function ==
  data: u input; y output
function y = fcn(u)
y=0.9089*u*u+0.19711*u;

== matlab function essai_echelon_volt/Refroidissement1/TEC1/MATLAB Function ==
  data: u input; y output
function y = fcn(u)
y=6.15*u;

== matlab function essai_echelon_volt/Chauffage1/Procédé/V2 2 R2 ==
  data: u input; y output
function y = fcn(u)

y = (((6300 + 3300)*5600*5)/(3300*u + 6300*1.8)) - 5600;

== matlab function essai_echelon_volt/Chauffage1/Procédé/V1 2 R1 ==
  data: u input; y output
function y = fcn(u)

y = (((3300 + 3300)*5600*5)/(3300*u + 3300*1.774)) - 5600;

== matlab function essai_echelon_volt/Chauffage1/Procédé/V3 2 R3 ==
  data: u input; y output
function y = fcn(u)

y = (((6300 + 3300)*5600*5)/(3300*u + 6300*1.79)) - 5600;

== matlab function essai_echelon_volt/Chauffage1/Procédé/R1 2 T1 ==
  data: u input; y output; T0_1 input
function y = fcn(u, T0_1)
y = (1/((log(u/10000)/4010)+(1/(T0_1+273.15))))-273.15;

== matlab function essai_echelon_volt/Chauffage1/Procédé/R2 2 T2 ==
  data: u input; y output; T0_2 input
function y = fcn(u, T0_2)

y = (1/((log(u/10000)/3984)+(T0_2+273.15)));

== matlab function essai_echelon_volt/Chauffage1/Procédé/R3 2 T3 ==
  data: u input; y output; T0_3 input
function y = fcn(u, T0_3)

y = (1/((log(u/10000)/3700)+(T0_3+273.15)))-273.15;
